simulink model "SimScape_PSFB_PCMC_HalfBridge_SRMode2"  (R2023b)
settings: Solver=VariableStepAuto  StartTime=0.0  StopTime=0.5  RelTol=1e-3
undefined symbols (not defined in the file): ADC_MaxCount, ADC_Vref, Gi_fb, L, Lm, n, Rload, Ro, Tcmpss, transformerCoupling
libraries: ee_lib x15, fl_lib x14, nesl_utility x11, simulink_extras x2, simulink x2, slpidlib x1, spspowerguiLib x1
(part 2 of 2)

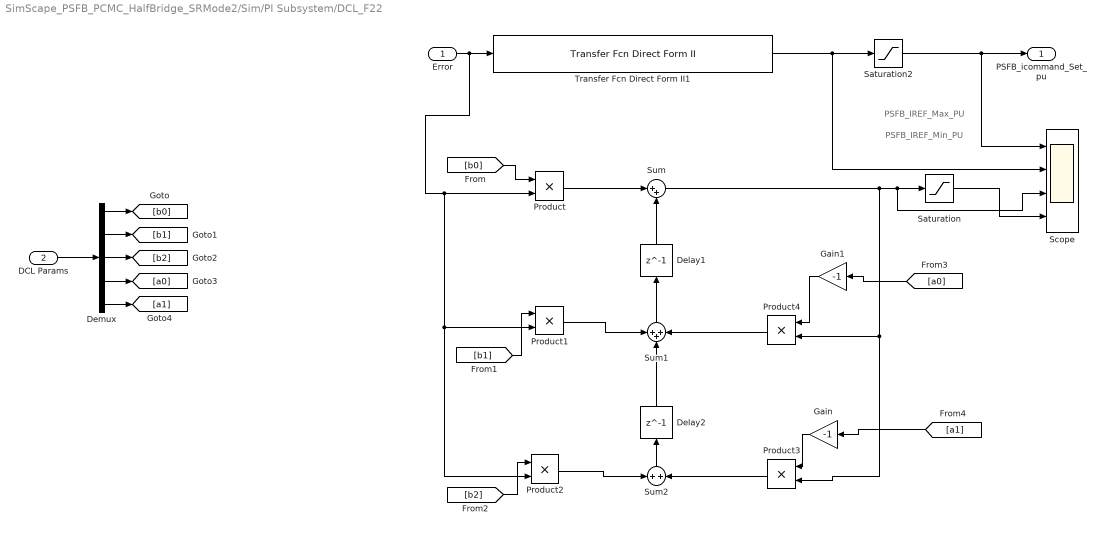
== system SimScape_PSFB_PCMC_HalfBridge_SRMode2/Sim/PI Subsystem/DCL_F22 ==
  note: PSFB_IREF_Min_PU
  note: PSFB_IREF_Max_PU
  Error : Inport
  DCL Params : Inport  Port=2
  Delay1 : Delay  DelayLength=1
  Delay2 : Delay  DelayLength=1
  Demux : Demux  Outputs=5
  Gain : Gain  Gain=-1
  Gain1 : Gain  Gain=-1
  Product{,1..4} (5 alike) : Product
  Saturation : Saturate  UpperLimit=0.9  LowerLimit=0.06
  Saturation2 : Saturate  UpperLimit=0.9  LowerLimit=0.06
  Scope : Scope  NumInputPorts=4
  Sum : Sum  Inputs=|++
  Sum1 : Sum  Inputs=+++
  Sum2 : Sum  Inputs=+|+
  Transfer Fcn Direct Form II1 : simulink/Additional Math & Discrete/Additional Discrete/Transfer Fcn Direct Form II  NumCoefVec=[14.0213636*2 -25.2978386*2 11.4016633*2]  DenCoefVec=[-1.8873439 0.8873439]  vinit=0.0  DoSatur=off
  PSFB_icommand_Set_pu : Outport
  wires:
  Delay1/1 -> Sum/2
  Delay2/1 -> Sum1/2
  Product3/1 -> Sum2/2
  Error/1 -> Product/2, Product2/2, Product1/2, Transfer Fcn Direct Form II1/1
  Product1/1 -> Sum1/1
  Sum2/1 -> Delay2/1
  Product/1 -> Sum/1
  Sum1/1 -> Delay1/1
  Product2/1 -> Sum2/1
  Product4/1 -> Sum1/3
  DCL Params/1 -> Demux/1
  Demux/1 -> [b0]
  Demux/5 -> [a1]
  Demux/4 -> [a0]
  Demux/3 -> [b2]
  Demux/2 -> [b1]
  [b0] -> Product/1
  [b2] -> Product2/1
  [b1] -> Product1/1
  Gain/1 -> Product3/1
  [a1] -> Gain/1
  Gain1/1 -> Product4/1
  [a0] -> Gain1/1
  Sum/1 -> Product4/2, Product3/2, Scope/3, Saturation/1
  Transfer Fcn Direct Form II1/1 -> Scope/2, Saturation2/1
  Saturation2/1 -> Scope/1, PSFB_icommand_Set_pu/1
  Saturation/1 -> Scope/4

== system SimScape_PSFB_PCMC_HalfBridge_SRMode2/Sim/PI Subsystem/PI Controller1 ==
  Error : Inport
  Kp : Inport  Port=2
  Ki : Inport  Port=3
  Gain : Gain  Gain=1/200e3
  PID Controller : slpidlib/PID Controller  Controller=PI  Form=Parallel  TimeDomain=Discrete-time  UseExternalTs=off  SampleTime=-1  IntegratorMethod=Forward Euler  FilterMethod=Forward Euler  ControllerParametersSource=external  P=1  I=1  UseKiTs=on  D=0  N=100  UseFilter=on  TunerSelectOption=Transfer Function Based (PID Tuner App)  InitialConditionSource=internal  InitialConditionForIntegrator=0  InitialConditionForFilter=0  DifferentiatorICPrevScaledInput=0  ExternalReset=none  TrackingMode=off  Kt=1  LimitOutput=on  SatLimitsSource=internal  UpperSaturationLimit=inf  LowerSaturationLimit=-inf  LinearizeAsGain=on  AntiWindupMode=none  Kb=1  LimitIntegrator=off  UpperIntegratorSaturationLimit=inf  LowerIntegratorSaturationLimit=-inf  POutMin=[]  POutMax=[]  IOutMin=[]  IOutMax=[]  DOutMin=[]  DOutMax=[]  NOutMin=[]  NOutMax=[]  SumOutMin=[]  SumOutMax=[]  SaturationOutMin=[]  SaturationOutMax=[]  PParamMin=[]  PParamMax=[]  IParamMin=[]  IParamMax=[]  DParamMin=[]  DParamMax=[]  NParamMin=[]  NParamMax=[]  KbParamMin=[]  KbParamMax=[]  KtParamMin=[]  KtParamMax=[]  KbOutMin=[]  KbOutMax=[]  KtOutMin=[]  KtOutMax=[]  IntegratorOutMin=[]  IntegratorOutMax=[]  FilterOutMin=[]  FilterOutMax=[]  SumI1OutMin=[]  SumI1OutMax=[]  SumI2OutMin=[]  SumI2OutMax=[]  SumI3OutMin=[]  SumI3OutMax=[]  SumI4OutMin=[]  SumI4OutMax=[]  SumDOutMin=[]  SumDOutMax=[]  DifferentiatorOutMin=[]  DifferentiatorOutMax=[]  FilterDiffOutCoefMin=[]  FilterDiffOutCoefMax=[]  ReciprocalOutMin=[]  ReciprocalOutMax=[]  SumDenOutMin=[]  SumDenOutMax=[]  SumNumOutMin=[]  SumNumOutMax=[]  DivideOutMin=[]  DivideOutMax=[]  UdiffTsProdOutMin=[]  UdiffTsProdOutMax=[]  NTsProdOutMin=[]  NTsProdOutMax=[]  UintegralTsProdOutMin=[]  UintegralTsProdOutMax=[]  UngainTsProdOutMin=[]  UngainTsProdOutMax=[]  ClampingZeroOutDataTypeStr=Inherit: Inherit via back propagation  ClampingZeroOutMin=[]  ClampingZeroOutMax=[]  FilterDenConstantOutDataTypeStr=Inherit: Inherit via back propagation  FilterDenConstantOutMin=[]  FilterDenConstantOutMax=[]  PCopyOutDataTypeStr=Inherit: Inherit via back propagation  PCopyOutMin=[]  PCopyOutMax=[]  NCopyOutDataTypeStr=Inherit: Inherit via back propagation  NCopyOutMin=[]  NCopyOutMax=[]  IntegratorContinuousStateAttributes=''  IntegratorStateMustResolveToSignalObject=off  IntegratorRTWStateStorageClass=Auto  FilterContinuousStateAttributes=''  FilterStateMustResolveToSignalObject=off  FilterRTWStateStorageClass=Auto  ParallelPVariant=ExternalParameters  IdealPVariant=Disabled  IVariant=ExternalParameters  DVariant=Disabled  IntegratorVariant=Discrete  SatVariant=Enabled  AWVariant=Passthrough  PCopyVariant=Disabled  TRVariant=Disabled  FdbkBlocksVariant=Forward  IdealPFdbkVariant=Disabled  SatFdbkVariant=Disabled  DerivativeFilterVariant=Disabled  NVariant=Disabled  NCopyVariant=Disabled_SignalSpec  FilterICVariant=Disabled  IntegratorICVariant=InternalICs  ExternalResetVariant=Disabled  TRSumVariant=Passthrough  SumFdbkVariant=Disabled  SumVariant=Sum_PI  TsampFilterVariant=InternalTs  TsampNgainVariant=Passthrough  TsampIntegralVariant=Disabled_SignalSpec  ExternalSaturationOutDataTypeStr=Inherit: Same as second input
  Saturation : Saturate  UpperLimit=1.0  LowerLimit=.05
  Scope : Scope  NumInputPorts=3
  Transfer Fcn Lead or Lag : simulink/Discrete/Transfer Fcn Lead or Lag  PoleZ=0.95  ZeroZ=0.75  ICPrevOutput=0.0  ICPrevInput=0.0  DoSatur=off
  Outp : Outport  VectorParamsAs1DForOutWhenUnconnected=off
  wires:
  Kp/1 -> PID Controller/2
  Error/1 -> Scope/3, PID Controller/1
  Saturation/1 -> Scope/1, Outp/1
  Ki/1 -> Gain/1
  PID Controller/1 -> Scope/2, Saturation/1
  Gain/1 -> PID Controller/3

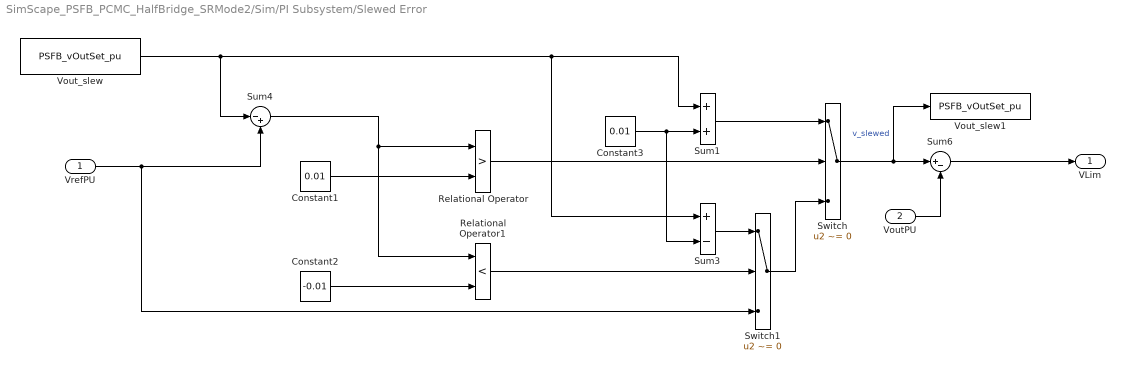
== system SimScape_PSFB_PCMC_HalfBridge_SRMode2/Sim/PI Subsystem/Slewed Error ==
  VrefPU : Inport
  VoutPU : Inport  Port=2
  Constant1 : Constant  Value=0.01  OutDataTypeStr=Inherit: Inherit via back propagation
  Constant2 : Constant  Value=-0.01  OutDataTypeStr=Inherit: Inherit via back propagation
  Constant3 : Constant  Value=0.01  OutDataTypeStr=Inherit: Inherit via back propagation
  Relational Operator : RelationalOperator  Operator=>  OutDataTypeStr=boolean  InputSameDT=off
  Relational Operator1 : RelationalOperator  Operator=<  OutDataTypeStr=boolean  InputSameDT=off
  Sum1 : Sum  RndMeth=Simplest  OutDataTypeStr=Inherit: Same as first input
  Sum3 : Sum  Inputs=+-  RndMeth=Simplest  OutDataTypeStr=Inherit: Same as first input
  Sum4 : Sum  Inputs=|-+  RndMeth=Simplest  OutDataTypeStr=Inherit: Same as first input
  Sum6 : Sum  Inputs=|+-  RndMeth=Simplest  OutDataTypeStr=Inherit: Same as first input
  Switch : Switch  Criteria=u2 ~= 0  RndMeth=Simplest  SaturateOnIntegerOverflow=off  InputSameDT=off
  Switch1 : Switch  Criteria=u2 ~= 0  RndMeth=Simplest  SaturateOnIntegerOverflow=off  InputSameDT=off
  Vout_slew : DataStoreRead  DataStoreName=PSFB_vOutSet_pu  IndexOptions=Index vector (dialog)  Indices=1  OutputSizes=1
  Vout_slew1 : DataStoreWrite  DataStoreName=PSFB_vOutSet_pu  IndexOptions=Index vector (dialog)  Indices=1  OutputSizes=1
  VLim : Outport  VectorParamsAs1DForOutWhenUnconnected=off
  wires:
  Sum4/1 -> Relational Operator1/1, Relational Operator/1
  Constant3/1 -> Sum3/2, Sum1/2
  Sum3/1 -> Switch1/1
  Relational Operator1/1 -> Switch1/2
  Switch1/1 -> Switch/3
  Sum1/1 -> Switch/1
  Relational Operator/1 -> Switch/2
  Constant1/1 -> Relational Operator/2
  VrefPU/1 -> Sum4/2, Switch1/3
  Vout_slew/1 -> Sum4/1, Sum3/1, Sum1/1
  Constant2/1 -> Relational Operator1/2
  Switch/1 -> Vout_slew1/1, Sum6/1  "v_slewed"
  VoutPU/1 -> Sum6/2
  Sum6/1 -> VLim/1
